simulink model "HyL_SV_new"  (R2015b)
settings: Solver=FixedStepAuto  StartTime=0.0  StopTime=3  FixedStep=1e-4  RelTol=1e-4
model workspace: external: MATLAB File C:\Users\Toshiba\Google Drive\Doutorado\Doutorado Sanduiche\IIT\Repositories\Job-IIT\03-Simulations\02-HyL\01-MATLAB_files\parameterInitialization.m (data not in the file)
values from neighbouring files (symbols this model uses):
  a1 = 0.3219    [param_JOB.m]
  a2 = 0.3218    [param_JOB.m]
  b1 = 0.045    [param_JOB.m]
  b2 = 0.045    [param_JOB.m]
  Lcyl = 0.280    (= 0.28)    [param_JOB.m]
  q0_0 = 0.75    [param_JOB.m]
  q1_0 = deg2rad(45)    [param_JOB.m]
  q1Max = deg2rad(70)    [param_JOB.m]
  q1Min = deg2rad(-50)    [param_JOB.m]
  q2_0 = deg2rad(-90)    [param_JOB.m]
  q2Max = deg2rad(-20)    [param_JOB.m]
  q2Min = deg2rad(-140)    [param_JOB.m]
undefined symbols (not defined in the file or in its folder): controllerCartSpace, Fpt, gcontact, gcPosVel, HyL_Job, referenceGenerator
libraries: simulink x5
settings Model: Creator=Toshiba  LastModifiedBy=Toshiba
settings SolverCC: AutoInsertRateTranBlk=on
settings DataIOCC: SaveFormat=Array
settings DebuggingCC: UnderspecifiedInitializationDetection=Classic  MergeDetectMultiDrivingBlocksExec=none  SolverPrmCheckMsg=warning  StateNameClashWarn=warning
settings HardwareCC: ProdBitPerPointer=32  ProdLargestAtomicFloat=None  ProdIntDivRoundTo=Undefined  ProdEndianess=Unspecified  ProdWordSize=32  ProdHWDeviceType=32-bit Generic
settings GRTTargetCC: GeneratePreprocessorConditionals=Disable all
settings ConfigComp: CovModelRefEnable=Off

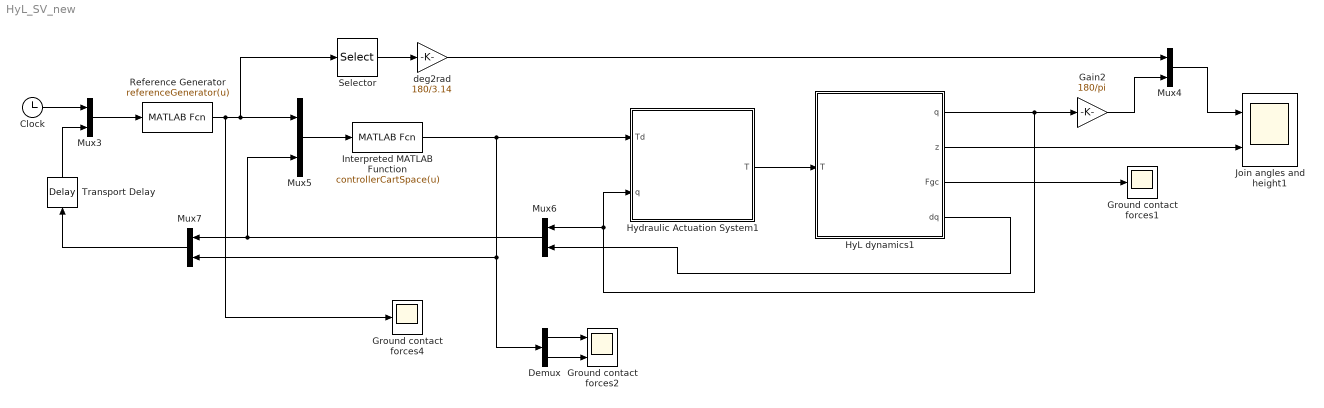
== system HyL_SV_new ==
  Clock : Clock
  Demux : Demux  Outputs=2
  Gain2 : Gain  Gain=180/pi
  Ground contact forces1 : Scope
  Ground contact forces2 : Scope  NumInputPorts=2
  Ground contact forces4 : Scope
  HyL dynamics1 : Subsystem
  Hydraulic Actuation System1 : Subsystem
  Interpreted MATLAB Function : MATLABFcn  MATLABFcn=controllerCartSpace(u)  OutputDimensions=2
  Join angles and height1 : Scope  NumInputPorts=2
  Mux{3..7} (5 alike) : Mux  Inputs=2
  Reference Generator : MATLABFcn  MATLABFcn=referenceGenerator(u)  OutputDimensions=4
  Selector : Selector  InputPortWidth=4  IndexOptions=Index vector (dialog)  Indices=[1 2]  OutputSizes=1
  Transport Delay : TransportDelay  DelayTime=0.0001
  deg2rad : Gain  Gain=180/3.14
  wires:
  Interpreted MATLAB Function/1 -> Hydraulic Actuation System1/1(Td), Demux/1, Mux7/2
  HyL dynamics1/1(q) -> Gain2/1, Hydraulic Actuation System1/2(q), Mux6/1
  HyL dynamics1/2(z) -> Join angles and height1/2
  Mux5/1 -> Interpreted MATLAB Function/1
  Gain2/1 -> Mux4/2
  Mux4/1 -> Join angles and height1/1
  HyL dynamics1/3(Fgc) -> Ground contact forces1/1
  HyL dynamics1/4(dq) -> Mux6/2
  Reference Generator/1 -> Ground contact forces4/1, Selector/1, Mux5/1
  Mux6/1 -> Mux5/2, Mux7/1
  Selector/1 -> deg2rad/1
  Mux7/1 -> Transport Delay/1
  Mux3/1 -> Reference Generator/1
  Transport Delay/1 -> Mux3/2
  Clock/1 -> Mux3/1
  Demux/1 -> Ground contact forces2/1
  Demux/2 -> Ground contact forces2/2
  deg2rad/1 -> Mux4/1
  Hydraulic Actuation System1/1(T) -> HyL dynamics1/1(T)

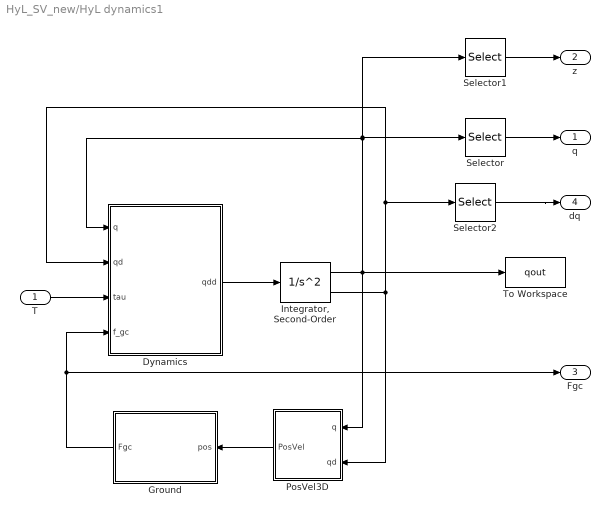
== system HyL_SV_new/HyL dynamics1 ==
  T : Inport
  Dynamics : Subsystem
  Ground : Subsystem
  "Integrator, Second-Order" : SecondOrderIntegrator  ICX=[q0_0;q1_0;q2_0]  LimitX=on  UpperLimitX=[inf; q1Max; q2Max]  LowerLimitX=[0; q1Min; q2Min]
  PosVel3D : Subsystem
  Selector : Selector  InputPortWidth=3  IndexOptions=Index vector (dialog)  Indices=[2 3]  OutputSizes=1
  Selector1 : Selector  InputPortWidth=3  IndexOptions=Index vector (dialog)  Indices=1  OutputSizes=1
  Selector2 : Selector  InputPortWidth=3  IndexOptions=Index vector (dialog)  Indices=[2 3]  OutputSizes=1
  To Workspace : ToWorkspace  VariableName=qout  SaveFormat=Timeseries  SampleTime=-1
  q : Outport
  z : Outport  Port=2
  Fgc : Outport  Port=3
  dq : Outport  Port=4
  wires:
  Dynamics/1(qdd) -> "Integrator, Second-Order"/1
  "Integrator, Second-Order"/1 -> Selector1/1, Selector/1, Dynamics/1(q), To Workspace/1, PosVel3D/1(q)
  "Integrator, Second-Order"/2 -> PosVel3D/2(qd), Dynamics/2(qd), Selector2/1
  Selector/1 -> q/1
  T/1 -> Dynamics/3(tau)
  Selector1/1 -> z/1
  PosVel3D/1(PosVel) -> Ground/1(pos)
  Ground/1(Fgc) -> Fgc/1, Dynamics/4(f_gc)
  Selector2/1 -> dq/1

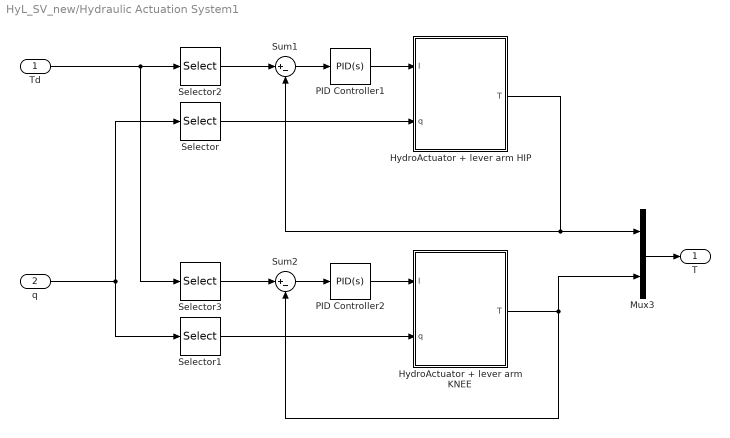
== system HyL_SV_new/Hydraulic Actuation System1 ==
  Td : Inport
  q : Inport  Port=2
  HydroActuator + lever arm HIP : Subsystem
  HydroActuator + lever arm KNEE : Subsystem
  Mux3 : Mux  Inputs=2
  PID Controller1 : simulink/Continuous/PID Controller  Controller=PID  TimeDomain=Continuous-time  SampleTime=-1  IntegratorMethod=Forward Euler  FilterMethod=Forward Euler  Form=Parallel  UseFilter=on  ControllerParametersSource=internal  P=200  I=0  D=5  N=100  InitialConditionSource=internal  InitialConditionForIntegrator=0  InitialConditionForFilter=0  ExternalReset=none  LimitOutput=off  UpperSaturationLimit=inf  LowerSaturationLimit=-inf  LinearizeAsGain=on  AntiWindupMode=none  Kb=1  TrackingMode=off  Kt=1  PParamMin=[]  PParamMax=[]  IParamMin=[]  IParamMax=[]  DParamMin=[]  DParamMax=[]  NParamMin=[]  NParamMax=[]  KbParamMin=[]  KbParamMax=[]  KtParamMin=[]  KtParamMax=[]  POutMin=[]  POutMax=[]  IOutMin=[]  IOutMax=[]  DOutMin=[]  DOutMax=[]  NOutMin=[]  NOutMax=[]  KbOutMin=[]  KbOutMax=[]  KtOutMin=[]  KtOutMax=[]  IntegratorOutMin=[]  IntegratorOutMax=[]  FilterOutMin=[]  FilterOutMax=[]  SumOutMin=[]  SumOutMax=[]  SumI1OutMin=[]  SumI1OutMax=[]  SumI2OutMin=[]  SumI2OutMax=[]  SumI3OutMin=[]  SumI3OutMax=[]  SumDOutMin=[]  SumDOutMax=[]  SaturationOutMin=[]  SaturationOutMax=[]  IntegratorContinuousStateAttributes=''  IntegratorStateMustResolveToSignalObject=off  IntegratorRTWStateStorageClass=Auto  FilterContinuousStateAttributes=''  FilterStateMustResolveToSignalObject=off  FilterRTWStateStorageClass=Auto  DifferentiatorICPrevScaledInput=0  DifferentiatorOutMin=[]  DifferentiatorOutMax=[]
  PID Controller2 : simulink/Continuous/PID Controller  Controller=PID  TimeDomain=Continuous-time  SampleTime=-1  IntegratorMethod=Forward Euler  FilterMethod=Forward Euler  Form=Parallel  UseFilter=on  ControllerParametersSource=internal  P=200  I=0  D=5  N=100  InitialConditionSource=internal  InitialConditionForIntegrator=0  InitialConditionForFilter=0  ExternalReset=none  LimitOutput=off  UpperSaturationLimit=inf  LowerSaturationLimit=-inf  LinearizeAsGain=on  AntiWindupMode=none  Kb=1  TrackingMode=off  Kt=1  PParamMin=[]  PParamMax=[]  IParamMin=[]  IParamMax=[]  DParamMin=[]  DParamMax=[]  NParamMin=[]  NParamMax=[]  KbParamMin=[]  KbParamMax=[]  KtParamMin=[]  KtParamMax=[]  POutMin=[]  POutMax=[]  IOutMin=[]  IOutMax=[]  DOutMin=[]  DOutMax=[]  NOutMin=[]  NOutMax=[]  KbOutMin=[]  KbOutMax=[]  KtOutMin=[]  KtOutMax=[]  IntegratorOutMin=[]  IntegratorOutMax=[]  FilterOutMin=[]  FilterOutMax=[]  SumOutMin=[]  SumOutMax=[]  SumI1OutMin=[]  SumI1OutMax=[]  SumI2OutMin=[]  SumI2OutMax=[]  SumI3OutMin=[]  SumI3OutMax=[]  SumDOutMin=[]  SumDOutMax=[]  SaturationOutMin=[]  SaturationOutMax=[]  IntegratorContinuousStateAttributes=''  IntegratorStateMustResolveToSignalObject=off  IntegratorRTWStateStorageClass=Auto  FilterContinuousStateAttributes=''  FilterStateMustResolveToSignalObject=off  FilterRTWStateStorageClass=Auto  DifferentiatorICPrevScaledInput=0  DifferentiatorOutMin=[]  DifferentiatorOutMax=[]
  Selector : Selector  InputPortWidth=2  IndexOptions=Index vector (dialog)  Indices=1  OutputSizes=1
  Selector1 : Selector  InputPortWidth=2  IndexOptions=Index vector (dialog)  Indices=2  OutputSizes=1
  Selector2 : Selector  InputPortWidth=2  IndexOptions=Index vector (dialog)  Indices=1  OutputSizes=1
  Selector3 : Selector  InputPortWidth=2  IndexOptions=Index vector (dialog)  Indices=2  OutputSizes=1
  Sum1 : Sum  Inputs=|+-
  Sum2 : Sum  Inputs=|+-
  T : Outport
  wires:
  Td/1 -> Selector3/1, Selector2/1
  q/1 -> Selector/1, Selector1/1
  Mux3/1 -> T/1
  HydroActuator + lever arm KNEE/1(T) -> Mux3/2, Sum2/2
  PID Controller2/1 -> HydroActuator + lever arm KNEE/1(I)
  Selector3/1 -> Sum2/1
  Selector1/1 -> HydroActuator + lever arm KNEE/2(q)
  Sum2/1 -> PID Controller2/1
  Selector2/1 -> Sum1/1
  Selector/1 -> HydroActuator + lever arm HIP/2(q)
  HydroActuator + lever arm HIP/1(T) -> Mux3/1, Sum1/2
  Sum1/1 -> PID Controller1/1
  PID Controller1/1 -> HydroActuator + lever arm HIP/1(I)

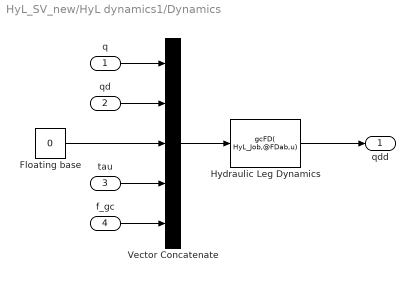
== system HyL_SV_new/HyL dynamics1/Dynamics ==
  q : Inport
  qd : Inport  Port=2
  tau : Inport  Port=3
  f_gc : Inport  Port=4
  Floating base : Constant  Value=0
  Hydraulic Leg Dynamics : MATLABFcn  MATLABFcn=gcFD( HyL_Job,@FDab,u)  OutputDimensions=[3 1]  OutputSignalType=real  Output1D=off
  Vector Concatenate : Concatenate  NumInputs=5
  qdd : Outport
  wires:
  Hydraulic Leg Dynamics/1 -> qdd/1
  Vector Concatenate/1 -> Hydraulic Leg Dynamics/1
  qd/1 -> Vector Concatenate/2
  q/1 -> Vector Concatenate/1
  f_gc/1 -> Vector Concatenate/5
  tau/1 -> Vector Concatenate/4
  Floating base/1 -> Vector Concatenate/3

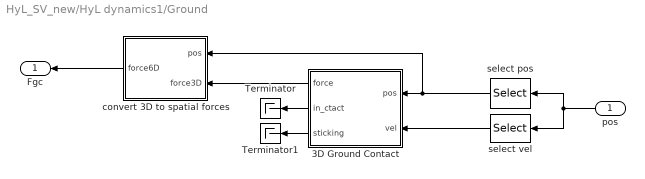
== system HyL_SV_new/HyL dynamics1/Ground ==
  pos : Inport
  3D Ground Contact : Subsystem  mask(3D Nonlinear Ground Contact with Friction){K=1e6, D=2000, mu=0.1, np=1}
      mask prompts: K "Stiffness (K)"; D "Damping (D)"; mu "Coefficient of Friction (mu)"; np "Number of Contact Points"
      mask help:
      | Given two 3xnp arrays containing contact-point positions and
      | velocities, calculate the 3xnp array of ground-reaction forces
      | acting on those points. Also calculate 1xnp boolean vectors
      | in_ctact (true if normal force >0) and sticking (true if inside
      | or on boundary of friction cone).  Zero-crossing detection is
      | enabled at both make/break contact and stick/slip transitions.
  Terminator : Terminator
  Terminator1 : Terminator
  convert 3D to spatial forces : Subsystem
  select pos : Selector  NumberOfDimensions=2  InputPortWidth=3  IndexOptions=Index vector (dialog),Select all  Indices=[1 2 3],1  OutputSizes=1,1
  select vel : Selector  NumberOfDimensions=2  InputPortWidth=3  IndexOptions=Index vector (dialog),Select all  Indices=[4 5 6],1  OutputSizes=1,1
  Fgc : Outport
  wires:
  select vel/1 -> 3D Ground Contact/2(vel)
  3D Ground Contact/1(force) -> convert 3D to spatial forces/2(force3D)
  3D Ground Contact/2(in_ctact) -> Terminator/1
  3D Ground Contact/3(sticking) -> Terminator1/1
  convert 3D to spatial forces/1(force6D) -> Fgc/1
  select pos/1 -> convert 3D to spatial forces/1(pos), 3D Ground Contact/1(pos)
  pos/1 -> select vel/1, select pos/1

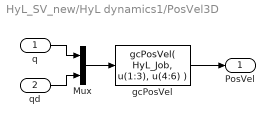
== system HyL_SV_new/HyL dynamics1/PosVel3D ==
  q : Inport
  qd : Inport  Port=2
  Mux : Mux  Inputs=2
  gcPosVel : MATLABFcn  MATLABFcn=gcPosVel( HyL_Job, u(1:3), u(4:6) )  OutputDimensions=[6 1]  OutputSignalType=real  Output1D=off
  PosVel : Outport
  wires:
  q/1 -> Mux/1
  qd/1 -> Mux/2
  Mux/1 -> gcPosVel/1
  gcPosVel/1 -> PosVel/1

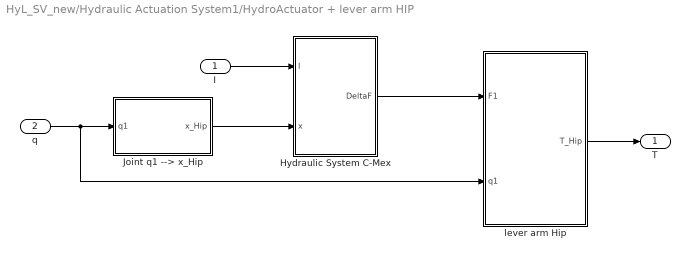
== system HyL_SV_new/Hydraulic Actuation System1/HydroActuator + lever arm HIP ==
  I : Inport
  q : Inport  Port=2
  Hydraulic System C-Mex : Subsystem
  "Joint q1 --> x_Hip  " : MATLAB Function  TreatAsAtomicUnit=on
  lever arm Hip : MATLAB Function  TreatAsAtomicUnit=on
  T : Outport
  wires:
  q/1 -> "Joint q1 --> x_Hip  "/1(q1), lever arm Hip/2(q1)
  lever arm Hip/1(T_Hip) -> T/1
  Hydraulic System C-Mex/1(DeltaF) -> lever arm Hip/1(F1)
  "Joint q1 --> x_Hip  "/1(x_Hip) -> Hydraulic System C-Mex/2(x)
  I/1 -> Hydraulic System C-Mex/1(I)

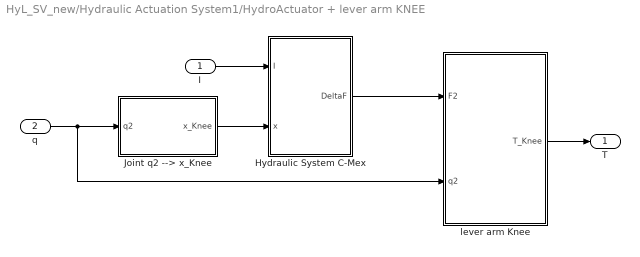
== system HyL_SV_new/Hydraulic Actuation System1/HydroActuator + lever arm KNEE ==
  I : Inport
  q : Inport  Port=2
  Hydraulic System C-Mex : Subsystem
  Joint q2 --> x_Knee : MATLAB Function  TreatAsAtomicUnit=on
  lever arm Knee : MATLAB Function  TreatAsAtomicUnit=on
  T : Outport
  wires:
  lever arm Knee/1(T_Knee) -> T/1
  Hydraulic System C-Mex/1(DeltaF) -> lever arm Knee/1(F2)
  q/1 -> lever arm Knee/2(q2), Joint q2 --> x_Knee/1(q2)
  Joint q2 --> x_Knee/1(x_Knee) -> Hydraulic System C-Mex/2(x)
  I/1 -> Hydraulic System C-Mex/1(I)

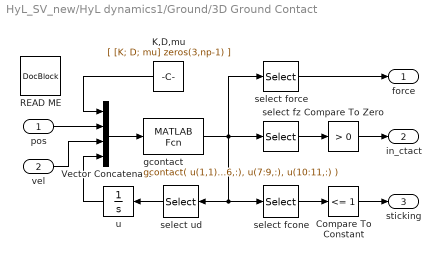
== system HyL_SV_new/HyL dynamics1/Ground/3D Ground Contact ==
  pos : Inport
  vel : Inport  Port=2
  Compare To Constant : simulink/Logic and Bit Operations/Compare To Constant  relop=<=  const=1  OutDataTypeStr=boolean
  Compare To Zero : simulink/Logic and Bit Operations/Compare To Zero  relop=>  OutDataTypeStr=boolean
  K,D,mu : Constant  Value=[ [K; D; mu] zeros(3,np-1) ]  VectorParams1D=off
  READ ME : simulink/Model-Wide Utilities/DocBlock  DocumentType=Text
      content=|
      | The constant block supplies the parameters K, D and mu to the function
      | gcontact.  This is necessary because K, D and mu are defined in the
      | workspace of this particular masked subsystem, but the executable
      | expression in the "MATLAB Function" block does not have access to this
      | workspace, so the symbols K, D and mu cannot appear directly in the
      | executable expression.
      |
      | The ">0" block and the "<=1" block both have zero-crossing enabled.  The
      | former detects transitions between contact and non-contact, whereas the
      | latter detects transitions between sticking (due to friction) and
      | slipping.  A point can be sticking only if it is also in contact.  A
      | zero-crossing event occurs whenever any one point makes a transition.
      |
      | The state variable, u, is a 2x(np) matrix containing the horizontal
      | component of the local ground deformation for each point.  This quantity
      | is used to calculate the tangential (i.e., frictional) component of the
      | ground reaction force.
      |
      | When a point loses contact, its associated state variable, u(:,i), decays
      | to zero with a time constant of D/K.  If this ratio is small then the
      | corresponding differential equation is fast, and it is necessary to use
      | small integration time steps.  For example, if K=1e6 and D=2000 then
      | D/K=0.002 and u(:,i) decays in proportion to exp(-500t).  Increasing K
      | makes the surface stiffer, and decreasing D/K makes it bouncier, but the
      | latter also makes the post-contact recovery faster.  The degree of
      | bounciness depends on the mass of the impacting body: a heavier body will
      | bounce more.
      |
      | To adapt this subsystem to work in 2D, the only things that change are the
      | row dimensions of various matrices.  You will have to alter the row
      | selections in the executable expression in the "MATLAB Function" block,
      | and also the dimensions of its output matrix, and you will have to change
      | the row selections in the various "select" blocks.
      |
      | For more information, see "The Simulink Ground Contact Model" in the
      | spatial_v2 documentation directory.
  Vector Concatenate : Concatenate  NumInputs=4  Mode=Multidimensional array
  gcontact : MATLABFcn  MATLABFcn=gcontact( u(1,1), u(2,1), u(3,1), u(4:6,:), u(7:9,:), u(10:11,:) )  OutputDimensions=[6 np]  OutputSignalType=real  Output1D=off
  select fcone : Selector  NumberOfDimensions=2  InputPortWidth=3  IndexOptions=Index vector (dialog),Select all  Indices=[6],1  OutputSizes=1,1
  select force : Selector  NumberOfDimensions=2  InputPortWidth=3  IndexOptions=Index vector (dialog),Select all  Indices=[1 2 3],1  OutputSizes=1,1
  select fz : Selector  NumberOfDimensions=2  InputPortWidth=3  IndexOptions=Index vector (dialog),Select all  Indices=[3],1  OutputSizes=1,1
  select ud : Selector  NumberOfDimensions=2  InputPortWidth=3  IndexOptions=Index vector (dialog),Select all  Indices=[4 5],1  OutputSizes=1,1
  u : Integrator
  force : Outport
  in_ctact : Outport  Port=2
  sticking : Outport  Port=3
  wires:
  Vector Concatenate/1 -> gcontact/1
  select ud/1 -> u/1
  gcontact/1 -> select fz/1, select ud/1, select fcone/1, select force/1
  select force/1 -> force/1
  select fz/1 -> Compare To Zero/1
  Compare To Zero/1 -> in_ctact/1
  select fcone/1 -> Compare To Constant/1
  Compare To Constant/1 -> sticking/1
  u/1 -> Vector Concatenate/4
  vel/1 -> Vector Concatenate/3
  pos/1 -> Vector Concatenate/2
  K,D,mu/1 -> Vector Concatenate/1

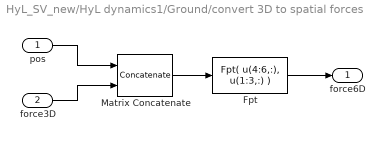
== system HyL_SV_new/HyL dynamics1/Ground/convert 3D to spatial forces ==
  pos : Inport
  force3D : Inport  Port=2
  Fpt : MATLABFcn  MATLABFcn=Fpt( u(4:6,:), u(1:3,:) )  OutputSignalType=real  Output1D=off
  Matrix Concatenate : Concatenate  Mode=Multidimensional array
  force6D : Outport
  wires:
  force3D/1 -> Matrix Concatenate/2
  pos/1 -> Matrix Concatenate/1
  Matrix Concatenate/1 -> Fpt/1
  Fpt/1 -> force6D/1

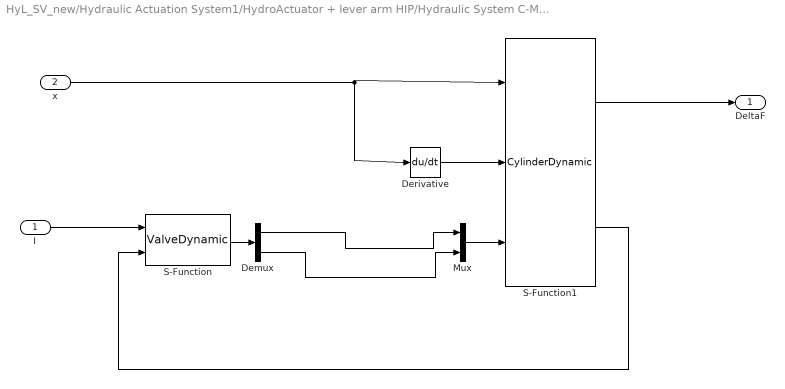
== system HyL_SV_new/Hydraulic Actuation System1/HydroActuator + lever arm HIP/Hydraulic System C-Mex ==
  I : Inport
  x : Inport  Port=2
  Demux : Demux  Outputs=2
  Derivative : Derivative
  Mux : Mux  Inputs=2
  S-Function : S-Function  FunctionName=ValveDynamic  Parameters=wn, E, In, Kva, Kvb, KvlkA, KvlkB, ps, pt,up_dz,lw_dz  SFunctionDeploymentMode=off  EnableBusSupport=off
  S-Function1 : S-Function  FunctionName=CylinderDynamic  Parameters=beta, V0A, V0B, Aa, Ab, L, fv, leak  SFunctionDeploymentMode=off  EnableBusSupport=off
  DeltaF : Outport
  wires:
  I/1 -> S-Function/1
  Derivative/1 -> S-Function1/2
  x/1 -> S-Function1/1, Derivative/1
  S-Function1/1 -> DeltaF/1
  S-Function1/2 -> S-Function/2
  S-Function/1 -> Demux/1
  Mux/1 -> S-Function1/3
  Demux/2 -> Mux/2
  Demux/1 -> Mux/1

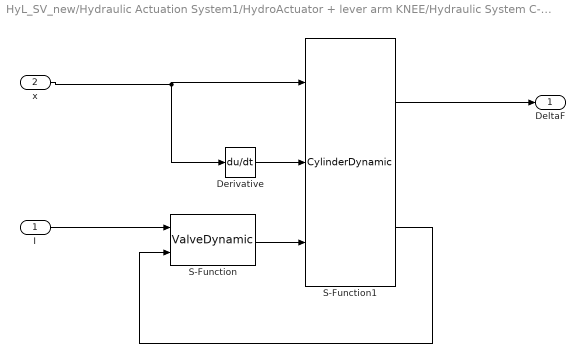
== system HyL_SV_new/Hydraulic Actuation System1/HydroActuator + lever arm KNEE/Hydraulic System C-Mex ==
  I : Inport
  x : Inport  Port=2
  Derivative : Derivative
  S-Function : S-Function  FunctionName=ValveDynamic  Parameters=wn, E, In, Kva, Kvb, KvlkA, KvlkB, ps, pt,up_dz,lw_dz  SFunctionDeploymentMode=off  EnableBusSupport=off
  S-Function1 : S-Function  FunctionName=CylinderDynamic  Parameters=beta, V0A, V0B, Aa, Ab, L, fv, leak  SFunctionDeploymentMode=off  EnableBusSupport=off
  DeltaF : Outport
  wires:
  I/1 -> S-Function/1
  Derivative/1 -> S-Function1/2
  x/1 -> S-Function1/1, Derivative/1
  S-Function1/2 -> S-Function/2
  S-Function/1 -> S-Function1/3
  S-Function1/1 -> DeltaF/1

== matlab function HyL_SV_new/Hydraulic Actuation System1/HydroActuator + lever arm HIP/Joint q1 --> x_Hip   ==
  data: a1 parameter; x_Hip output; b1 parameter; e11 parameter; e12 parameter; Lcyl parameter; q1 input
% HIP joint space - HIP Lin Actuator

function x_Hip = fcn(a1,b1,e11,e12,Lcyl,q1)
%#codegen

%Hip
ang1 = pi/2 - q1 + e11 - e12; 
c1 = sqrt(a1^2 + b1^2 - 2*a1*b1*cos(ang1));

x_Hip = c1-Lcyl;

== matlab function HyL_SV_new/Hydraulic Actuation System1/HydroActuator + lever arm HIP/lever arm Hip ==
  data: a1 parameter; T_Hip output; b1 parameter; e11 parameter; e12 parameter; F1 input; q1 input
% Lever Arm calculation
% HIP

function T_Hip = fcn(a1,b1,e11,e12,F1,q1)
%#codegen

%Hip
ang1 = pi/2 - q1 + e11 - e12; 
c1 = sqrt(a1^2 + b1^2 - 2*a1*b1*cos(ang1));
L1 = a1*sin(acos((a1^2+c1^2-b1^2)/(2*a1*c1)));
T_Hip = F1*L1;

== matlab function HyL_SV_new/Hydraulic Actuation System1/HydroActuator + lever arm KNEE/Joint q2 --> x_Knee ==
  data: a2 parameter; x_Knee output; b2 parameter; e21 parameter; e22 parameter; Lcyl parameter; q2 input
% KNEE joint space - KNEE Lin Actuator

function x_Knee = fcn(a2,b2,e21,e22,Lcyl,q2)
%#codegen

%Knee
ang2 = pi + q2 - e21 - e22;
c2 = sqrt(a2^2 + b2^2 - 2*a2*b2*cos(ang2));
x_Knee = c2-Lcyl;

== matlab function HyL_SV_new/Hydraulic Actuation System1/HydroActuator + lever arm KNEE/lever arm Knee ==
  data: a2 parameter; T_Knee output; b2 parameter; e21 parameter; e22 parameter; F2 input; q2 input
% Lever Arm calculation
% KNEE

function T_Knee = fcn(a2,b2,e21,e22,F2,q2)
%#codegen

%Knee
ang2 = pi + q2 - e21 - e22;
c2 = sqrt(a2^2 + b2^2 - 2*a2*b2*cos(ang2));
L2 = a2*sin(acos((a2^2+c2^2-b2^2)/(2*a2*c2)));
T_Knee = F2*L2;
